simulink model "AD7403"  (R2014b)
settings: Solver=FixedStepDiscrete  StartTime=0.0  StopTime=0.0022  RelTol=1e-3
InitFcn:
  | Fclk = 20e6
settings Model: Creator=tmacleod  LastModifiedBy=tmacleod
settings SolverCC: AutoInsertRateTranBlk=on

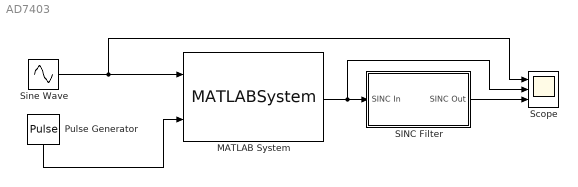
== system AD7403 ==
  MATLAB System : MATLABSystem  System=AD7403_sysobj  SimulateUsing=Interpreted execution  Mode=Modulator  Fclk=20e6
      mask Type: AD7403_sysobj
      mask Display:
      | disp('AD7403');
      | port_label('input',1,'in (V)');
      | port_label('input',2,'MCLKIN');
      | port_label('output',1,'out (Bit)');
  Pulse Generator : DiscretePulseGenerator  PulseType=Time based  Period=1.0/Fclk*2  PulseWidth=50  mask{Fclk=Fclk}
  SINC Filter : Subsystem  mask{Order=3, M=256, Fclk=20e6}
      mask prompts: M "Decimation"
      mask TypeOptions Order: 1 | 2 | 3 | 4
  Scope : Scope  NumInputPorts=3
      settings: YMin=-5~-5~-5  YMax=5~5~5
  Sine Wave : Sin  Amplitude=0.32  Frequency=2*pi*1000  SampleTime=0
  wires:
  Pulse Generator/1 -> MATLAB System/2
  MATLAB System/1 -> Scope/2, SINC Filter/1(SINC In)
  SINC Filter/1(SINC Out) -> Scope/3
  Sine Wave/1 -> Scope/1, MATLAB System/1

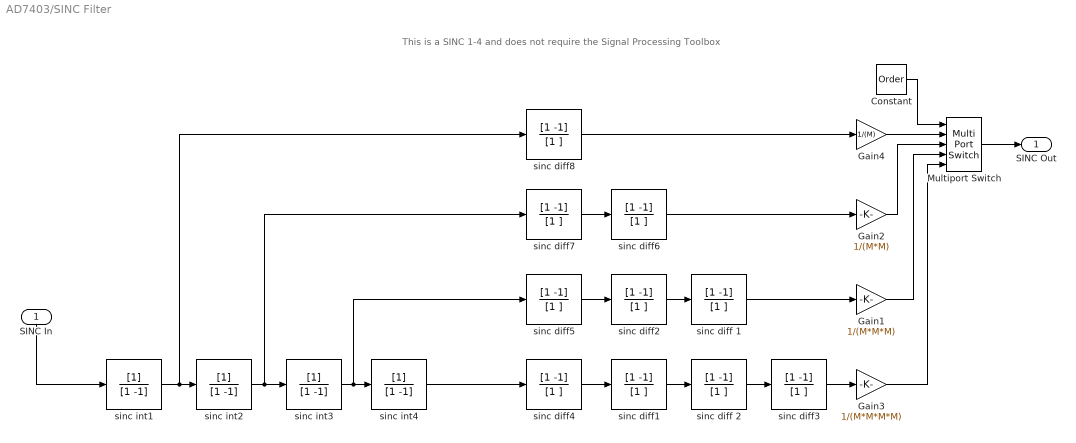
== system AD7403/SINC Filter ==
  note: This is a SINC 1-4 and does not require the Signal Processing Toolbox
  SINC In : Inport
  Constant : Constant  Value=Order
  Gain1 : Gain  Gain=1/(M*M*M)  SaturateOnIntegerOverflow=on  OutDataTypeStr=Inherit: Same as input  ParamDataTypeStr=Inherit: Same as input
  Gain2 : Gain  Gain=1/(M*M)  SaturateOnIntegerOverflow=on  OutDataTypeStr=Inherit: Same as input  ParamDataTypeStr=Inherit: Same as input
  Gain3 : Gain  Gain=1/(M*M*M*M)  SaturateOnIntegerOverflow=on  OutDataTypeStr=Inherit: Same as input  ParamDataTypeStr=Inherit: Same as input
  Gain4 : Gain  Gain=1/(M)  SaturateOnIntegerOverflow=on  OutDataTypeStr=Inherit: Same as input  ParamDataTypeStr=Inherit: Same as input
  Multiport Switch : MultiPortSwitch  DataPortOrder=Specify indices  DataPortIndices={1,2,3,4}
  sinc diff 1 : DiscreteFilter  Numerator=[1 -1]  Denominator=[1 ]  SampleTime=M/Fclk
  sinc diff 2 : DiscreteFilter  Numerator=[1 -1]  Denominator=[1 ]  SampleTime=M/Fclk
  sinc diff{1..8} (8 alike) : DiscreteFilter  Numerator=[1 -1]  Denominator=[1 ]  SampleTime=M/Fclk
  sinc int{1..4} (4 alike) : DiscreteFilter  Denominator=[1 -1]  SampleTime=1/Fclk
  SINC Out : Outport
  wires:
  sinc diff 2/1 -> sinc diff3/1
  sinc diff3/1 -> Gain3/1
  sinc diff1/1 -> sinc diff 2/1
  sinc int1/1 -> sinc diff8/1, sinc int2/1
  SINC In/1 -> sinc int1/1
  sinc int2/1 -> sinc int3/1, sinc diff7/1
  sinc diff2/1 -> sinc diff 1/1
  sinc diff 1/1 -> Gain1/1
  Constant/1 -> Multiport Switch/1
  Multiport Switch/1 -> SINC Out/1
  sinc int3/1 -> sinc diff5/1, sinc int4/1
  sinc diff4/1 -> sinc diff1/1
  sinc int4/1 -> sinc diff4/1
  sinc diff5/1 -> sinc diff2/1
  sinc diff7/1 -> sinc diff6/1
  sinc diff8/1 -> Gain4/1
  sinc diff6/1 -> Gain2/1
  Gain3/1 -> Multiport Switch/5
  Gain1/1 -> Multiport Switch/4
  Gain2/1 -> Multiport Switch/3
  Gain4/1 -> Multiport Switch/2
